simulink library "v2x_baseband"  (R2021b)
settings: Solver=VariableStepAuto  StartTime=0.0  StopTime=10.0  RelTol=1e-3
undefined symbols (not defined in the file or in its folder): rsgenpoly
libraries: commblkcod2 x2, commsequence2 x2, v2x_type_conv x2, visionstatistics x1
settings Model: Creator=jacob  LastModifiedBy=ryans

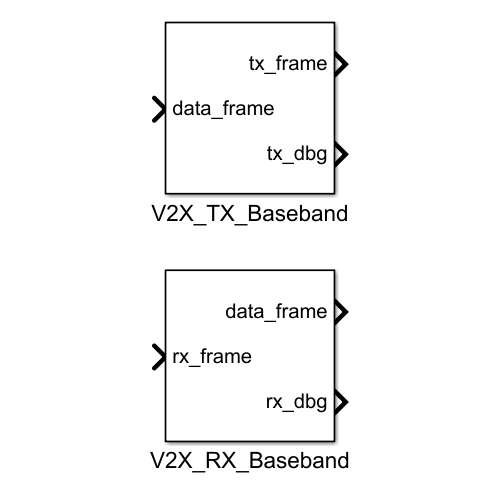
[thumbnail: Simulink's stored preview of the top-level diagram]
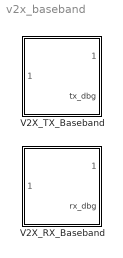
== system v2x_baseband ==
  V2X_RX_Baseband : Subsystem
      mask init:
      | ini = v2x_baseband_init();
  V2X_TX_Baseband : Subsystem
      mask init:
      | ini = v2x_baseband_init();

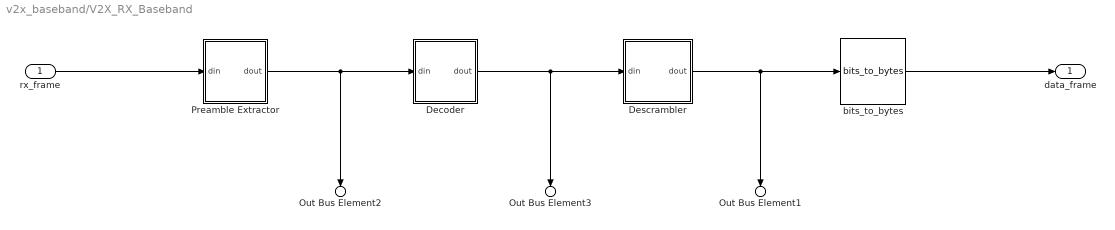
== system v2x_baseband/V2X_RX_Baseband ==
  rx_frame : Inport
  Decoder : Subsystem
  Descrambler : Subsystem
  Preamble Extractor : Subsystem
  bits_to_bytes : v2x_type_conv/bits_to_bytes  bit_frame_len=bb_ini.pkt.data_len
  data_frame : Outport
  Out Bus Element2 : Outport  Port=2  PortName=rx_dbg  Element=dec_in
  Out Bus Element3 : Outport  Port=2  PortName=rx_dbg  Element=descr_in
  Out Bus Element1 : Outport  Port=2  PortName=rx_dbg  Element=bits_out
  wires:
  bits_to_bytes/1 -> data_frame/1
  rx_frame/1 -> Preamble Extractor/1(din)
  Preamble Extractor/1(dout) -> Decoder/1(din), Out Bus Element2/1
  Decoder/1(dout) -> Out Bus Element3/1, Descrambler/1(din)
  Descrambler/1(dout) -> Out Bus Element1/1, bits_to_bytes/1

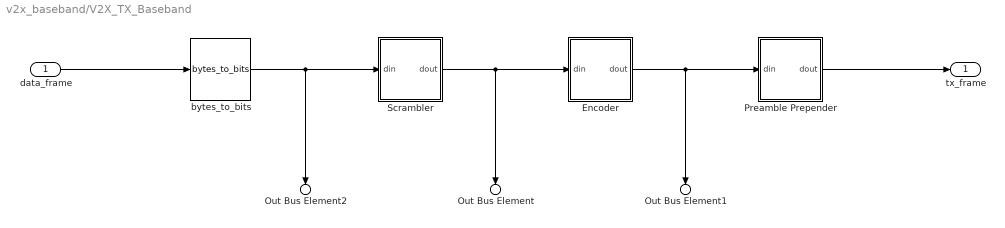
== system v2x_baseband/V2X_TX_Baseband ==
  data_frame : Inport
  Encoder : Subsystem
  Preamble Prepender : Subsystem
  Scrambler : Subsystem
  bytes_to_bits : v2x_type_conv/bytes_to_bits  SystemSampleTime=-1  VariantActivationTime=update diagram  Latency=0  AutoFrameSizeCalculation=off
  tx_frame : Outport
  Out Bus Element2 : Outport  Port=2  PortName=tx_dbg  Element=bits_in
  Out Bus Element : Outport  Port=2  PortName=tx_dbg  Element=scramb_out
  Out Bus Element1 : Outport  Port=2  PortName=tx_dbg  Element=enc_out
  wires:
  bytes_to_bits/1 -> Out Bus Element2/1, Scrambler/1(din)
  Preamble Prepender/1(dout) -> tx_frame/1
  data_frame/1 -> bytes_to_bits/1
  Scrambler/1(dout) -> Out Bus Element/1, Encoder/1(din)
  Encoder/1(dout) -> Out Bus Element1/1, Preamble Prepender/1(din)

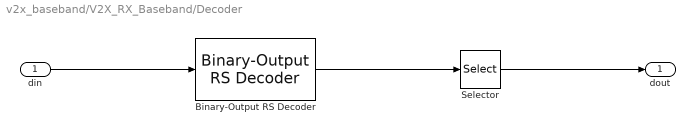
== system v2x_baseband/V2X_RX_Baseband/Decoder ==
  din : Inport
  Binary-Output RS Decoder : commblkcod2/Binary-Output RS Decoder  n=ini.enc.n  k=ini.enc.k  specShortening=off  shortenedK=3  specGenPoly=off  genPoly=rsgenpoly(7, 3, [], [], 'double')  specPrimPoly=off  prPoly='X^3 + X + 1'  specPuncture=off  punctVec=[ones(2,1); zeros(2,1)]  specErasurePort=off  showNumErr=off  outDType=Same as input
      settings: SourceProductBaseCode=CM
  Selector : Selector  InputPortWidth=ini.pkt.data_len + ini.enc.extra_bits  IndexOptions=Starting index (dialog)  Indices=1  OutputSizes=ini.pkt.data_len
  dout : Outport
  wires:
  Selector/1 -> dout/1
  Binary-Output RS Decoder/1 -> Selector/1
  din/1 -> Binary-Output RS Decoder/1

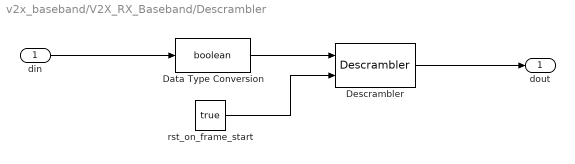
== system v2x_baseband/V2X_RX_Baseband/Descrambler ==
  din : Inport
  Data Type Conversion : DataTypeConversion  OutDataTypeStr=boolean
  Descrambler : commsequence2/Descrambler  M=2  poly=ini.scramb.tap  iniStaSource=Dialog Parameter  ini_sta=ini.scramb.seed  resetViaPort=on
      settings: SourceProductBaseCode=CM
  rst_on_frame_start : Constant  Value=true  SampleTime=-1
  dout : Outport
  wires:
  rst_on_frame_start/1 -> Descrambler/2
  Descrambler/1 -> dout/1
  din/1 -> Data Type Conversion/1
  Data Type Conversion/1 -> Descrambler/1

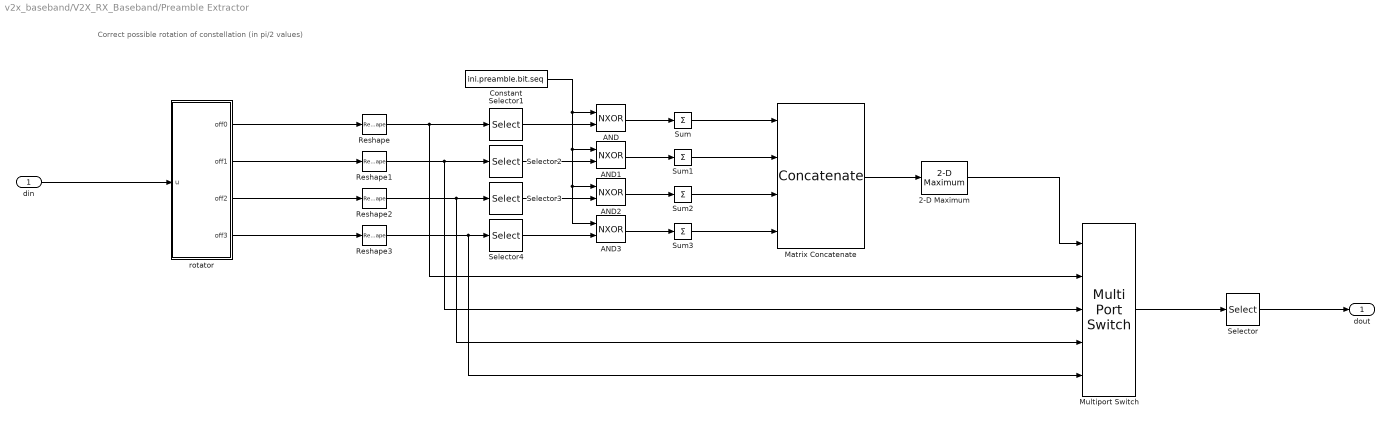
== system v2x_baseband/V2X_RX_Baseband/Preamble Extractor ==
  note: Correct possible rotation of constellation (in pi/2 values)
  din : Inport
  2-D Maximum : visionstatistics/2-D Maximum  fcn=Index  reset=None  indexBase=One  operateOver=Each column  Dimension=1  colComp=on  operation=maximum  accumLastDataTypeStr=Inherit: Same as product output  roiEnable=off  roiType=Rectangles  roiPortion=Entire ROI  roiOutput=Individual statistics for each ROI  roiFlag=off  roundingMode=Floor  overflowMode=off  accumDataTypeStr=Inherit: Same as product output
      settings: SourceProductBaseCode=VP
  AND{,1..3} (4 alike) : Logic  Operator=NXOR  AllPortsSameDT=off  OutDataTypeStr=boolean
  Constant : Constant  Value=ini.preamble.bit.seq  VectorParams1D=off  SampleTime=-1
  Matrix Concatenate : Concatenate  NumInputs=4  Mode=Multidimensional array
  Multiport Switch : MultiPortSwitch  Inputs=4  DiagnosticForDefault=Warning
  Reshape{,1..3} (4 alike) : Reshape  OutputDimensionality=Column vector (2-D)
  Selector : Selector  InputPortWidth=ini.intfc.rx_bit_len  IndexOptions=Starting index (dialog)  Indices=ini.preamble.bit.len + 1  OutputSizes=ini.enc.len
  Selector{1..4} (4 alike) : Selector  InputPortWidth=ini.intfc.rx_bit_len  IndexOptions=Starting index (dialog)  Indices=1  OutputSizes=ini.preamble.bit.len
  Sum{,1..3} (4 alike) : Sum  Inputs=+
  rotator : MATLAB Function  TreatAsAtomicUnit=on
  dout : Outport
  wires:
  Multiport Switch/1 -> Selector/1
  2-D Maximum/1 -> Multiport Switch/1
  Selector/1 -> dout/1
  Matrix Concatenate/1 -> 2-D Maximum/1
  Sum3/1 -> Matrix Concatenate/4
  Sum2/1 -> Matrix Concatenate/3
  Sum1/1 -> Matrix Concatenate/2
  Sum/1 -> Matrix Concatenate/1
  AND3/1 -> Sum3/1
  AND2/1 -> Sum2/1
  AND1/1 -> Sum1/1
  AND/1 -> Sum/1
  Selector2/1 -> AND1/2
  Selector3/1 -> AND2/2
  Selector4/1 -> AND3/2
  Constant/1 -> AND/1, AND1/1, AND2/1, AND3/1
  Selector1/1 -> AND/2
  Reshape3/1 -> Selector4/1, Multiport Switch/5
  Reshape2/1 -> Selector3/1, Multiport Switch/4
  Reshape1/1 -> Selector2/1, Multiport Switch/3
  Reshape/1 -> Multiport Switch/2, Selector1/1
  rotator/2(off1) -> Reshape1/1
  rotator/4(off3) -> Reshape3/1
  rotator/3(off2) -> Reshape2/1
  rotator/1(off0) -> Reshape/1
  din/1 -> rotator/1(u)

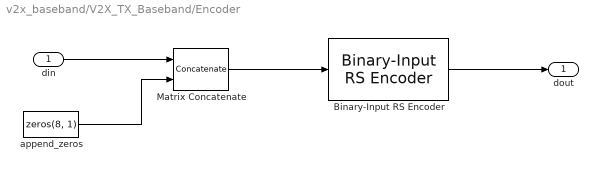
== system v2x_baseband/V2X_TX_Baseband/Encoder ==
  din : Inport
  Binary-Input RS Encoder : commblkcod2/Binary-Input RS Encoder  n=ini.enc.n  k=ini.enc.k  specShortening=off  shortenedK=3  specGenPoly=off  genPoly=rsgenpoly(7, 3, [], [], 'double')  specPrimPoly=off  prPoly='X^3 + X + 1'  specPuncture=off  punctVec=[ones(2,1); zeros(2,1)]  outDType=Same as input
      settings: SourceProductBaseCode=CM
  Matrix Concatenate : Concatenate  Mode=Multidimensional array
  append_zeros : Constant  Value=zeros(8, 1)  VectorParams1D=off  OutDataTypeStr=boolean  SampleTime=-1
  dout : Outport
  wires:
  Matrix Concatenate/1 -> Binary-Input RS Encoder/1
  append_zeros/1 -> Matrix Concatenate/2
  din/1 -> Matrix Concatenate/1
  Binary-Input RS Encoder/1 -> dout/1

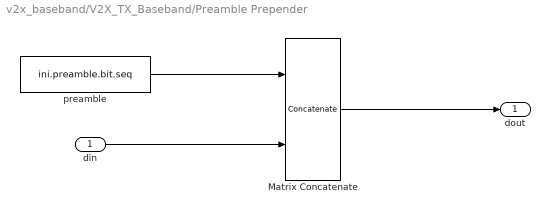
== system v2x_baseband/V2X_TX_Baseband/Preamble Prepender ==
  din : Inport
  Matrix Concatenate : Concatenate  Mode=Multidimensional array
  preamble : Constant  Value=ini.preamble.bit.seq  VectorParams1D=off  OutDataTypeStr=boolean  SampleTime=-1
  dout : Outport
  wires:
  preamble/1 -> Matrix Concatenate/1
  din/1 -> Matrix Concatenate/2
  Matrix Concatenate/1 -> dout/1

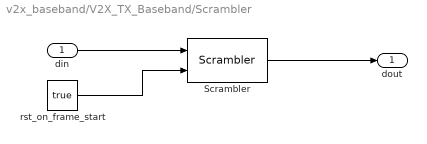
== system v2x_baseband/V2X_TX_Baseband/Scrambler ==
  din : Inport
  Scrambler : commsequence2/Scrambler  M=2  poly=ini.scramb.tap  iniStaSource=Dialog Parameter  ini_sta=ini.scramb.seed  resetViaPort=on
      settings: SourceProductBaseCode=CM
  rst_on_frame_start : Constant  Value=true  SampleTime=-1
  dout : Outport
  wires:
  rst_on_frame_start/1 -> Scrambler/2
  Scrambler/1 -> dout/1
  din/1 -> Scrambler/1

== matlab function v2x_baseband/V2X_RX_Baseband/Preamble Extractor/rotator ==
  data: u input; off0 output; off1 output; off2 output; off3 output
function [off0, off1, off2, off3] = rotator(u)
    % 0 rotation
    off0 = u;

    % pi/2 rotation
    temp1 = reshape(u, 2, length(u)/2);
    for n = 1:length(u)/2
        if ~temp1(1, n) && ~temp1(2, n) % 00 -> 01
            temp1(1, n) = false;
            temp1(2, n) = true;
        elseif ~temp1(1, n) && temp1(2, n) % 01 -> 11
            temp1(1, n) = true;
            temp1(2, n) = true;
        elseif temp1(1, n) && temp1(2, n) % 11 -> 10
            temp1(1, n) = true;
            temp1(2, n) = false;
        else % 10 -> 00
            temp1(1, n) = false;
            temp1(2, n) = false;
        end
    end
    off1 = temp1(:);

    % pi rotation
    off2 = not(u);

    % 3pi/2 rotation
    temp3 = reshape(u, 2, length(u)/2);
    for n = 1:length(u)/2
        if ~temp3(1, n) && ~temp3(2, n) % 00 -> 10
            temp3(1, n) = true;
            temp3(2, n) = false;
        elseif ~temp3(1, n) && temp3(2, n) % 01 -> 00
            temp3(1, n) = false;
            temp3(2, n) = false;
        elseif temp3(1, n) && temp3(2, n) % 11 -> 01
            temp3(1, n) = false;
            temp3(2, n) = true;
        else % 10 -> 11
            temp3(1, n) = true;
            temp3(2, n) = true;
        end
    end
    off3 = temp3(:);
end
